simulink model "Closedloop_PI"  (R2018a)
settings: Solver=VariableStepAuto  StartTime=0.0  StopTime=300  MaxStep=0.01  RelTol=1e-3  EnableMultiTasking=on
values from neighbouring files (symbols this model uses):
  a11 = -Cr/Jr    (= -0.000211148648649)    [Run_img_closedloop.m]
  a12 = 0    [Run_img_closedloop.m]
  a13 = -1/Jr    (= -3.37837837838e-07)    [Run_img_closedloop.m]
  a21 = 0    [Run_img_closedloop.m]
  a22 = -Cg/Jg    (= -0.000942755863941)    [Run_img_closedloop.m]
  a23 = 1/ng/Jg    (= 0.000214347948375)    [Run_img_closedloop.m]
  a31 = Kls-Cls*Cr/Jr    (= 559978.885135)    [Run_img_closedloop.m]
  a32 = (Cls*Cg/Jg-Kls)/ng    (= -6365.09662267)    [Run_img_closedloop.m]
  a33 = -Cls*(Jr+ng^2*Jg)/(ng^2*Jg*Jr)    (= -0.277457913694)    [Run_img_closedloop.m]
  b11 = 1/Jr    (= 3.37837837838e-07)    [Run_img_closedloop.m]
  b12 = 0    [Run_img_closedloop.m]
  b21 = 0    [Run_img_closedloop.m]
  b22 = -1/Jg    (= -0.0188551172788)    [Run_img_closedloop.m]
  b31 = Cls/Jr    (= 0.0337837837838)    [Run_img_closedloop.m]
  b32 = Cls/ng/Jg    (= 21.4347948375)    [Run_img_closedloop.m]
  beta_opt = 2    [Run_img_closedloop.m]
  Cp = xlsread(filename)    [Run_img_closedloop.m]
  lambda_opt = 7.1    [Run_img_closedloop.m]
  R = 35    [Run_img_closedloop.m]
  Rho = 1.225    [Run_img_closedloop.m]
  vf = xlsread(filename)    [Run_img_closedloop.m]
libraries: simulink x1
settings Model: Creator=alino  LastModifiedBy=alino
settings DataIOCC: LimitDataPoints=on
settings OptimizationCC: LifeSpan=inf
settings DebuggingCC: AllowSymbolicDim=off  SFUnexpectedBacktrackingDiag=warning  SFNoUnconditionalDefaultTransitionDiag=warning  SFExecutionAtInitializationDiag=none
settings ModelReferenceCC: PropagateSignalLabelsOutOfModel=off
settings CodeAppCC: StateflowObjectComments=on
settings GRTTargetCC: TargetLangStandard=C89/C90 (ANSI)
settings ConfigComp: CovMetricSettings=dw  CovHtmlReporting=on  CovSaveCumulativeToWorkspaceVar=on  CovSaveSingleToWorkspaceVar=on  CovExternalEMLEnable=off

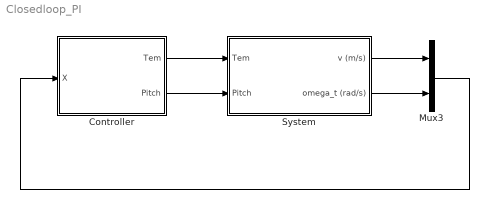
== system Closedloop_PI ==
  Controller : Subsystem
  Mux3 : Mux  Inputs=2
  System : Subsystem
  wires:
  Mux3/1 -> Controller/1(X)
  Controller/1(Tem) -> System/1(Tem)
  Controller/2(Pitch) -> System/2(Pitch)
  System/2(omega_t (rad/s)) -> Mux3/2
  System/1(v (m/s)) -> Mux3/1

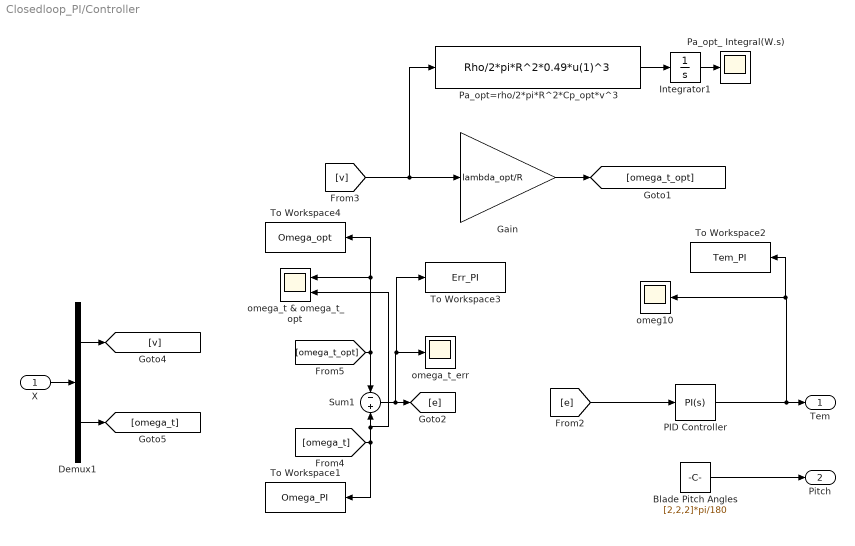
== system Closedloop_PI/Controller ==
  X : Inport
  Blade Pitch Angles : Constant  Value=[2,2,2]*pi/180
  Demux1 : Demux  Outputs=2
  Gain : Gain  Gain=lambda_opt/R
  Integrator1 : Integrator
  PID Controller : simulink/Continuous/PID Controller  Controller=PI  TimeDomain=Continuous-time  SampleTime=-1  IntegratorMethod=Forward Euler  FilterMethod=Forward Euler  Form=Parallel  UseFilter=on  ControllerParametersSource=internal  P=6711  I=1555  D=3902.663  N=249.734444057219  InitialConditionSource=internal  InitialConditionForIntegrator=0  InitialConditionForFilter=0  ExternalReset=none  LimitOutput=off  UpperSaturationLimit=inf  LowerSaturationLimit=-inf  LinearizeAsGain=on  AntiWindupMode=none  Kb=1  TrackingMode=off  Kt=1  PParamMin=[]  PParamMax=[]  IParamMin=[]  IParamMax=[]  DParamMin=[]  DParamMax=[]  NParamMin=[]  NParamMax=[]  KbParamMin=[]  KbParamMax=[]  KtParamMin=[]  KtParamMax=[]  POutMin=[]  POutMax=[]  IOutMin=[]  IOutMax=[]  DOutMin=[]  DOutMax=[]  NOutMin=[]  NOutMax=[]  KbOutMin=[]  KbOutMax=[]  KtOutMin=[]  KtOutMax=[]  IntegratorOutMin=[]  IntegratorOutMax=[]  FilterOutMin=[]  FilterOutMax=[]  SumOutMin=[]  SumOutMax=[]  SumI1OutMin=[]  SumI1OutMax=[]  SumI2OutMin=[]  SumI2OutMax=[]  SumI3OutMin=[]  SumI3OutMax=[]  SumDOutMin=[]  SumDOutMax=[]  SaturationOutMin=[]  SaturationOutMax=[]  IntegratorContinuousStateAttributes=''  IntegratorStateMustResolveToSignalObject=off  IntegratorRTWStateStorageClass=Auto  FilterContinuousStateAttributes=''  FilterStateMustResolveToSignalObject=off  FilterRTWStateStorageClass=Auto  DifferentiatorICPrevScaledInput=0  DifferentiatorOutMin=[]  DifferentiatorOutMax=[]  FilterDiffOutCoefMin=[]  FilterDiffOutCoefMax=[]  SumDenOutMin=[]  SumDenOutMax=[]  SumNumOutMin=[]  SumNumOutMax=[]  ReciprocalOutMin=[]  ReciprocalOutMax=[]  DivideOutMin=[]  DivideOutMax=[]  TunerSelectOption=Transfer Function Based (PID Tuner App)
  Pa_opt=rho/2*pi*R^2*Cp_opt*v^3 : Fcn  Expr=Rho/2*pi*R^2*0.49*u(1)^3
  Pa_opt_ Integral(W.s) : Scope
  Sum1 : Sum  Inputs=-+
  To Workspace1 : ToWorkspace  VariableName=Omega_PI  SaveFormat=Timeseries  SampleTime=-1
  To Workspace2 : ToWorkspace  VariableName=Tem_PI  SaveFormat=Timeseries  SampleTime=-1
  To Workspace3 : ToWorkspace  VariableName=Err_PI  SaveFormat=Timeseries  SampleTime=-1
  To Workspace4 : ToWorkspace  VariableName=Omega_opt  SaveFormat=Timeseries  SampleTime=-1
  omeg10 : Scope
  omega_t & omega_t_opt : Scope  NumInputPorts=2
  omega_t_err : Scope
  Tem : Outport
  Pitch : Outport  Port=2
  wires:
  X/1 -> Demux1/1
  Demux1/1 -> [v]
  Demux1/2 -> [omega_t]
  Blade Pitch Angles/1 -> Pitch/1
  PID Controller/1 -> To Workspace2/1, omeg10/1, Tem/1
  [v] -> Pa_opt=rho/2*pi*R^2*Cp_opt*v^3/1, Gain/1
  Gain/1 -> [omega_t_opt]
  Sum1/1 -> To Workspace3/1, omega_t_err/1, [e]
  [omega_t_opt] -> To Workspace4/1, omega_t & omega_t_opt/1, Sum1/1
  [omega_t] -> To Workspace1/1, omega_t & omega_t_opt/2, Sum1/2
  [e] -> PID Controller/1
  Integrator1/1 -> Pa_opt_ Integral(W.s)/1
  Pa_opt=rho/2*pi*R^2*Cp_opt*v^3/1 -> Integrator1/1

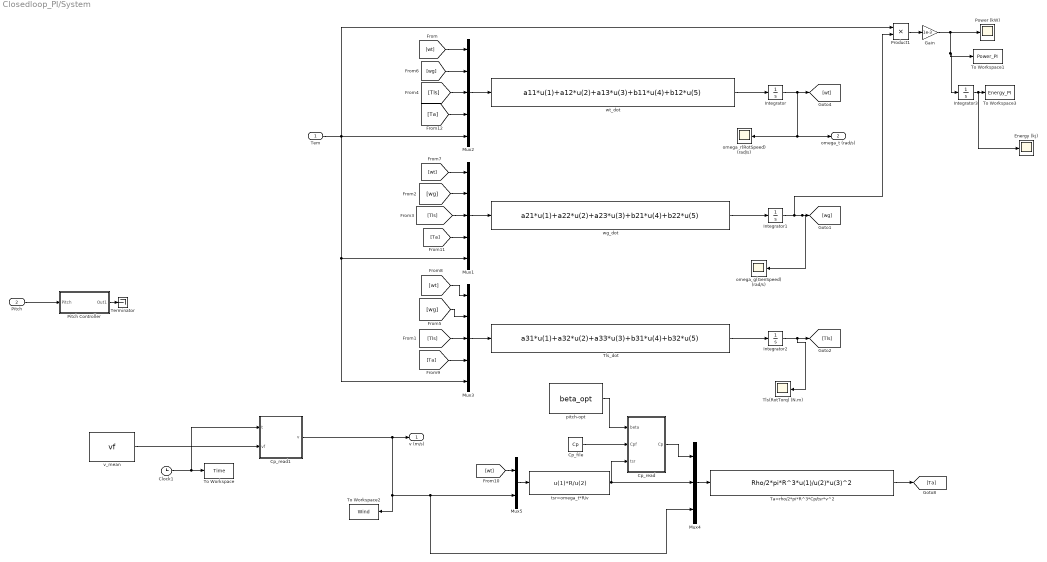
== system Closedloop_PI/System ==
  Tem : Inport
  Pitch : Inport  Port=2
  Clock1 : Clock
  Cp_file : Constant  Value=Cp
  Cp_read : MATLAB Function  TreatAsAtomicUnit=on
  Cp_read1 : MATLAB Function  TreatAsAtomicUnit=on
  Energy (kj) : Scope
  Gain : Gain  Gain=1e-3
  Integrator : Integrator  InitialCondition=1
  Integrator1 : Integrator  InitialCondition=1
  Integrator2 : Integrator
  Integrator3 : Integrator  InitialCondition=1
  Mux1 : Mux  Inputs=5
  Mux2 : Mux  Inputs=5
  Mux3 : Mux  Inputs=5
  Mux4 : Mux  Inputs=3
  Mux5 : Mux  Inputs=2
  Pitch Controller : Subsystem
  Power (kW) : Scope
  Product1 : Product
  Ta=rho/2*pi*R^3*Cp/tsr*v^2 : Fcn  Expr=Rho/2*pi*R^3*u(1)/u(2)*u(3)^2
  Terminator : Terminator
  Tls(RotTorq) (N.m) : Scope
  Tls_dot : Fcn  Expr=a31*u(1)+a32*u(2)+a33*u(3)+b31*u(4)+b32*u(5)
  To Workspace : ToWorkspace  VariableName=Time  SampleTime=-1
  To Workspace1 : ToWorkspace  VariableName=Power_PI  SaveFormat=Timeseries  SampleTime=-1
  To Workspace2 : ToWorkspace  VariableName=Wind  SaveFormat=Timeseries  SampleTime=-1
  To Workspace3 : ToWorkspace  VariableName=Energy_PI  SaveFormat=Timeseries  SampleTime=-1
  omega_g(GenSpeed) (rad/s) : Scope
  omega_r(RotSpeed) (rad/s) : Scope
  pitch-opt : Constant  Value=beta_opt
  tsr=omega_t*R/v : Fcn  Expr=u(1)*R/u(2)
  v_mean : Constant  Value=vf
  wg_dot : Fcn  Expr=a21*u(1)+a22*u(2)+a23*u(3)+b21*u(4)+b22*u(5)
  wt_dot : Fcn  Expr=a11*u(1)+a12*u(2)+a13*u(3)+b11*u(4)+b12*u(5)
  v (m/s) : Outport
  omega_t (rad/s) : Outport  Port=2
  wires:
  Clock1/1 -> Cp_read1/1(t), To Workspace/1
  Integrator/1 -> omega_t (rad/s)/1, omega_r(RotSpeed) (rad/s)/1, [wt]
  Integrator2/1 -> Tls(RotTorq) (N.m)/1, [Tls]
  Pitch/1 -> Pitch Controller/1(Pitch)
  Mux2/1 -> wt_dot/1
  Mux1/1 -> wg_dot/1
  Mux3/1 -> Tls_dot/1
  wt_dot/1 -> Integrator/1
  [wt] -> Mux2/1
  wg_dot/1 -> Integrator1/1
  Tls_dot/1 -> Integrator2/1
  [wt] -> Mux3/1
  [wg] -> Mux1/2
  [Tls] -> Mux3/3
  [Tls] -> Mux1/3
  [Tls] -> Mux2/3
  [wg] -> Mux3/2
  [wg] -> Mux2/2
  [wt] -> Mux1/1
  Pitch Controller/1(Out1) -> Terminator/1
  Mux4/1 -> Ta=rho/2*pi*R^3*Cp/tsr*v^2/1
  Cp_read1/1(v) -> To Workspace2/1, Mux4/3, Mux5/2, v (m/s)/1
  Mux5/1 -> tsr=omega_t*R/v/1
  [wt] -> Mux5/1
  tsr=omega_t*R/v/1 -> Mux4/2, Cp_read/3(tsr)
  Ta=rho/2*pi*R^3*Cp/tsr*v^2/1 -> [Ta]
  Cp_read/1(Cp) -> Mux4/1
  Cp_file/1 -> Cp_read/2(Cpf)
  pitch-opt/1 -> Cp_read/1(beta)
  [Ta] -> Mux3/4
  [Ta] -> Mux1/4
  [Ta] -> Mux2/4
  v_mean/1 -> Cp_read1/2(vf)
  Integrator1/1 -> omega_g(GenSpeed) (rad/s)/1, [wg], Product1/2
  Tem/1 -> Product1/1, Mux3/5, Mux1/5, Mux2/5
  Product1/1 -> Gain/1
  Gain/1 -> Power (kW)/1, Integrator3/1, To Workspace1/1
  Integrator3/1 -> Energy (kj)/1, To Workspace3/1

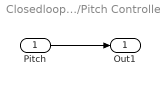
== system Closedloop_PI/System/Pitch Controller ==
  Pitch : Inport
  Out1 : Outport
  wires:
  Pitch/1 -> Out1/1

== matlab function Closedloop_PI/System/Cp_read1 ==
  data: t input; v output; vf input
function v = fcn(t,vf)
    v=vf(floor(2*t)+1);
end

== matlab function Closedloop_PI/System/Cp_read ==
  data: beta input; Cpf input; Cp output; tsr input
function Cp = fcn(beta,Cpf,tsr)

    if (tsr>19) || (beta>90) || (tsr<1) 
        Cp=0;
    else
    beta1=floor(beta)+1;
    tsr1=floor(tsr*10);
    beta2=beta1+1;
    tsr2=tsr1+1;
    betap=beta-floor(beta);
    tsrp=tsr*10-floor(tsr*10);
    Cp1=Cpf(beta1,tsr1)+betap*(Cpf(beta2,tsr1)-Cpf(beta1,tsr1));
    Cp2=Cpf(beta1,tsr2)+betap*(Cpf(beta2,tsr2)-Cpf(beta1,tsr2));
    Cp=tsrp*(Cp2-Cp1)+Cp1;
    end
end
